simulink model "Basic_Drone_Waypoint_part"  (R2024a)
settings: Solver=FixedStepAuto  StartTime=0.0  StopTime=inf  FixedStep=0.1  RelTol=1e-3
undefined symbols (not defined in the file): Angle, Axis, DiscIntNeverNeededParam, gray
libraries: robotcorelib x10, slpidlib x4, eeGeneralControl x4, uavutilslib x1
settings Model: Creator=Sasha  LastModifiedBy=user

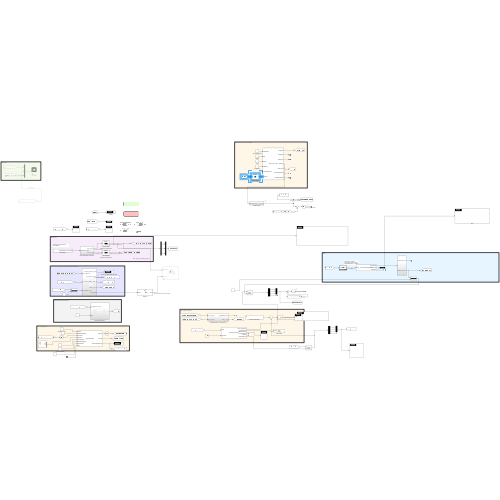
[thumbnail: Simulink's stored preview of the top-level diagram]
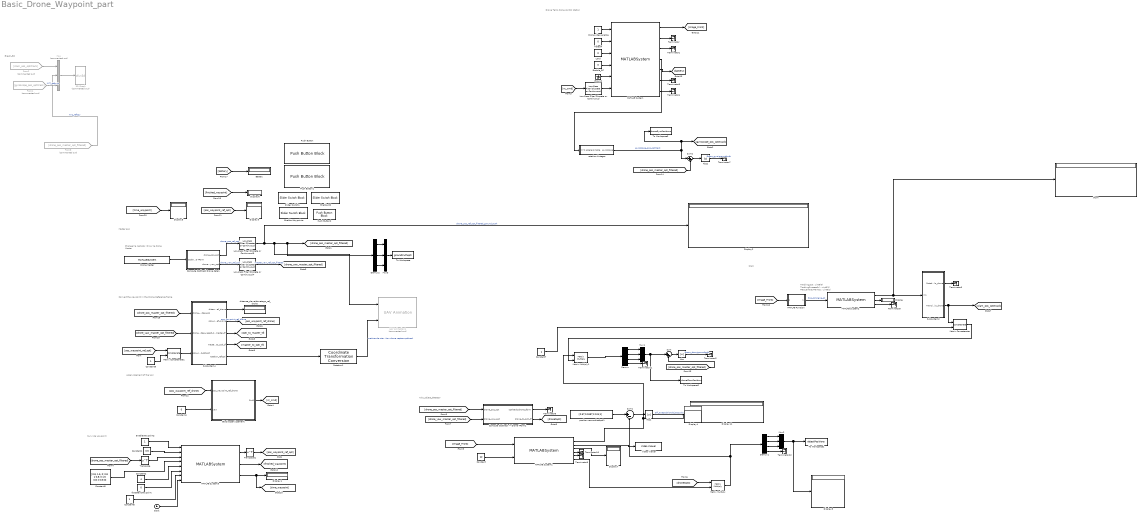
== system Basic_Drone_Waypoint_part ==
  note: Suivi de waypoint
  note: Drone Tello drone control station
  note: Asservissement of the UAV
  note: TrackingLost : uint8(0)
      | TrackingSuccessful : uint8(1)
      | FrequentKeyFrames : uint8(2)
  note: Slam
  note: Graph_3D
  note: Changer le rigibody ID sur le drone Master
  note: Master pos
  note: Convert the waypoint in the Drone Reference frame
  note: Yolo_object_detector
  3D Graph : S-Function  Commented=on  LoadFcn=if exist('sfun3d','file'), sfun3d([],[],[],'LoadBlock'); end  FunctionName=sfun3d  Parameters=ax,T,np,cp,gd,ls,mk,mx,hd,tb  SFunctionDeploymentMode=off  EnableBusSupport=off  mask(3D Graph){np=3, ax=[-5 5 -5 5 -5 5], mx=1e4, T=-1, cp=[3 2 1], gd=on, hd=off, tb=on, ls=-, mk=none}
      mask prompts: np "Number of moving points (lines)"; ax "Range: [xmin xmax  ymin ymax zmin zmax]"; mx "Max number of points in each line"; T "Sampling Time"; cp "Camera position (use [0 0 1] for 2D XY view)"; gd "Grid (on|off)"; hd "HeadMarkers (on|off)"; tb "Toolbar (on|off)"; ls "LineStyle"; mk "LineMarker"
      mask help:
      | This block plots the position of several points in the XYZ space. The input contains the coordinates of all the points (x1,y1,z1,x2,y2,z2,...).
      | The number of moving points (lines), the XYZ ranges, sampling time, camera position, and grid (among other things) can be set as mask parameters.
      settings: CopyFcn=if exist('sfun3d','file'), sfun3d([],[],[],'CopyBlock'); end  DeleteFcn=if exist('sfun3d','file'), sfun3d([],[],[],'DeleteBlock'); end  NameChangeFcn=if exist('sfun3d','file'), sfun3d([],[],[],'NameChange'); end
      mask Help:
      | This block plots the position of several points in the XYZ space. The input contains the coordinates of all the points (x1,y1,z1,x2,y2,z2,...).
      | The number of moving points (lines), the XYZ ranges, sampling time, camera position, and grid (among other things) can be set as mask parameters.
      mask TypeOptions ls: - | -- | : | -. | none
      mask TypeOptions mk: none | . | + | o | * | x | square | diamond | v | ^ | > | < | pentagram | hexagram
      mask Display: plot([.05 .95 .95 .05 .05],[.45 .45 .95 .95 .45], 0.5+cos(0:0.1:2*pi)*0.3,0.7+sin(0:0.1:2*pi)*0.2)
  Abs : Abs  SaturateOnIntegerOverflow=off
  Abs1 : Abs  SaturateOnIntegerOverflow=off
  Abs2 : Abs  SaturateOnIntegerOverflow=off
  Battery : Display
  "Block asservissement " : Subsystem
  Clock : Clock
  "Compute Optitrack -> Drone TForm1" : Subsystem
  Compute Optitrack Drone data1 : Subsystem
  Constant : Constant  Value=12
  Constant1 : Constant  Value=0.5
  Constant2 : Constant  Value=4
  Constant3 : Constant  Value=[0.8, 1.5, 0; 0.8 1 0.8; 0 1.5 0.8; 0 0.8 0]
  Constant4 : Constant  Value=0
  Constant5 : Constant
  Constant6 : Constant
  Constant7 : Constant
  Demux : Demux
  Demux1 : Demux
  Demux2 : Demux  Outputs=3
  Display{,1..8,11} (10 alike) : Display
  Drone Master : MATLABSystem  System=OptilinkSystem  HostIP=10.147.125.15  ClientIP=10.147.125.15  RigidbodyID=2  SimulateUsing=Interpreted execution
      mask Type: OptilinkSystem
      mask Display:
      | disp('OptilinkSystem');
      | port_label('output',1,'Drones data');
  Dronevideo enable : Constant
  Enable RC : SliderSwitchBlock
      settings: Values={{'Off', 'On'}, [0 1]}
  Enable Waypoints : SliderSwitchBlock
      settings: Values={{'Off', 'On'}, [0 1]}
  Enable_RC : Constant  Value=0
  From1 : From  Commented=on  GotoTag=gyroscope_pos_optitrack
  From2 : From  Commented=on  GotoTag=slam_pos_optitrack
  From8 : From  Commented=on  GotoTag=drone_pos_master_opt_filtered
  Ground : Ground
  Land : Constant  Value=0
  Low-Pass Filter (Discrete or Continuous) : eeGeneralControl/Low-Pass Filter (Discrete or Continuous)  K=1  T=1  B=inf  A=-inf  init_option=Inherited from block input  x0=0  Ts=-1
  Low-Pass Filter (Discrete or Continuous)4 : eeGeneralControl/Low-Pass Filter (Discrete or Continuous)  K=1  T=1.5  B=inf  A=-inf  init_option=Inherited from block input  x0=0  Ts=-1
  Low-Pass Filter (Discrete or Continuous)5 : eeGeneralControl/Low-Pass Filter (Discrete or Continuous)  K=1  T=1.5  B=inf  A=-inf  init_option=Inherited from block input  x0=0  Ts=-1
  MATLAB Function : MATLAB Function  TreatAsAtomicUnit=on
  MATLAB System : MATLABSystem  System=Tello_drone_control  droneIP=127.0.0.1  SimulateUsing=Interpreted execution
      mask Type: Tello_drone_control
      mask Display:
      | disp('Tello_drone_control');
      | port_label('input',1,'enableVideo');
      | port_label('input',2,'tkoff');
      | port_label('input',3,'landing');
      | port_label('input',4,'enableRC');
      | port_label('input',5,'cmdVideoDirection');
      | port_label('input',6,'rcspeeds');
      | port_label('output',1,'imageFront');
      | port_label('output',2,'imageDown');
      | port_label('output',3,'Eulerangles');
      | port_label('output',4,'speedXYZ');
      | port_label('output',5,'batteryLevel');
      | port_label('output',6,'currentVideoDirection');
      | port_label('output',7,'hasTakenOffStatus');
  MATLAB System1 : MATLABSystem  System=Yolo_Object_Detector  SimulateUsing=Interpreted execution
      mask Type: Yolo_Object_Detector
      mask Display:
      | disp('Yolo_Object_Detector');
      | port_label('input',1,'Image');
      | port_label('input',2,'degreecam');
      | port_label('output',1,'Tform_camtodrone');
      | port_label('output',2,'AnnotatedImage');
      | port_label('output',3,'BBoxDimensions');
      | port_label('output',4,'CamCoordinates');
      | port_label('output',5,'posecam');
      | port_label('output',6,'posecamtodrone');
  MATLAB System2 : MATLABSystem  System=MonoVisualSLAMSystem  FocalLength=[ 878, 883.00 ]  PrincipalPoint=[ 488, 363 ]  ImageSize=[ 720, 960 ]  ScaleFactor=1.2  NumLevels=6  MaxNumPoints=200  SkipMaxFrames=10  TrackFeatureRange=[ 50, 120 ]  LoopClosureThreshold=50  Verbose=false  ThreadLevel=3  SimulateUsing=Code generation
      mask Type: MonoVisualSLAMSystem
      mask Display:
      | disp('MonoVisualSLAMSystem');
      | port_label('input',1,'Image');
      | port_label('output',1,'Camera Pose');
      | port_label('output',2,'Tracking Lost');
      | port_label('output',3,'XYZ Points');
  MATLAB System3 : MATLABSystem  System=WaypointManager  SimulateUsing=Code generation
      mask Type: WaypointManager
      mask Display:
      | disp('WaypointManager');
      | port_label('input',1,'enable');
      | port_label('input',2,'lookaheadDistance');
      | port_label('input',3,'currentPos');
      | port_label('input',4,'waypoints');
      | port_label('input',5,'numWaypoints');
      | port_label('input',6,'forceNextWaypoint');
      | port_label('input',7,'requiredTime');
      | port_label('input',8,'time');
      | port_label('output',1,'waypoint');
      | port_label('output',2,'finished');
      | port_label('output',3,'elapsedTimeWaypoint');
  Matrix Concatenate : Concatenate  ConcatenateDimension=2
  Matrix Concatenate1 : Concatenate  ConcatenateDimension=2
  Matrix Multiply : Product  Multiplication=Matrix(*)
  Matrix Multiply1 : Product  Multiplication=Matrix(*)
  Mux : Mux  Commented=on  Inputs=3
  Mux1 : Mux  Inputs=3
  Mux2 : Mux  Inputs=3
  Mux3 : Mux  Inputs=3
  Push Button : PushButtonBlock  ButtonText=Décoler  OffValue=0.000000
  Push Button1 : PushButtonBlock  ButtonText=Atterir  OffValue=0.000000
  Push Button2 : PushButtonBlock  ButtonText=Next waypoint  OffValue=0.000000
  Rotation1 : robotcorelib/Coordinate Transformation Conversion  InputRepresentation=Rotation Matrix  InputEulerSequence=XYZ  ShowTrVecInputPort=off  OutputRepresentation=Quaternion  OutputEulerSequence=ZYX  ShowTrVecOutputPort=off  SimulateUsing=Code generation
      settings: LibrarySourceBlock=uavutilslib/Coordinate Transformation Conversion
  Slider Switch1 : SliderSwitchBlock
      settings: Values={{'Off', 'On'}, [0 1]}
  Subsystem2 : Subsystem
  Subsystem4 : Subsystem
  Sum : Sum  Inputs=|+-
  Sum1 : Sum  Inputs=|+-
  Sum2 : Sum  Inputs=|+-
  Takeoff : Constant  Value=0
  Terminator{,1..12} (13 alike) : Terminator
  To Workspace : ToWorkspace  VariableName=groundtruthopti  SampleTime=-1
  To Workspace1 : ToWorkspace  VariableName=objectPositions  SampleTime=-1
  To Workspace2 : ToWorkspace  VariableName=droneSlamPositions  SampleTime=-1
  To Workspace3 : ToWorkspace  VariableName=droneGyroPositions  SampleTime=-1
  Transpose : Math  Operator=transpose
  Transpose1 : Math  Operator=transpose
  UAV Animation1 : uavutilslib/UAV Animation  Commented=on  UAVType=Multirotor  UAVSize=1  InertialZDirection=Down  SampleTime=-1
  Video Viewer : VideoViewer  colormapValue=gray(256)  FigPos=[231 1060 894 657]
  distance_slave/slavetogo_ref_drone : Display
  enableWaypoints : Constant
  forceNextWaypoint : Constant  Value=0
  posiiton camordirefopti1 : Constant  Value=[0.57;0.1597;2.124;1]
  rotation+integer : Subsystem
  tform : Display
  wires:
  Land/1 -> MATLAB System/3
  Takeoff/1 -> MATLAB System/2
  Enable_RC/1 -> MATLAB System/4
  [rc_cmd] -> Low-Pass Filter (Discrete or Continuous)/1
  Low-Pass Filter (Discrete or Continuous)/1 -> MATLAB System/6
  MATLAB System/6 -> Terminator3/1
  MATLAB System2/2 -> Display/1
  MATLAB System2/1 -> tform/1, Subsystem2/1(In1)
  From8/1 -> Mux/2  "XYZ_refopy"
  Mux/1 -> 3D Graph/1
  From1/1 -> Mux/3  "XYZ_refgyro"
  MATLAB System/1 -> [Image_Front]
  MATLAB System/2 -> Terminator/1
  Dronevideo enable/1 -> MATLAB System/1
  MATLAB System/3 -> Terminator1/1
  MATLAB System/5 -> [battery]
  MATLAB System/7 -> Terminator4/1
  rotation+integer/1(gyroscope) -> [gyroscope_pos_optitrack], To Workspace3/1, Sum2/1  "gyroscope_pos_optitrack"
  Compute Optitrack Drone data1/1(drone_pos_opt) -> Low-Pass Filter (Discrete or Continuous)5/1  "drone_pos_ref_opt"
  Low-Pass Filter (Discrete or Continuous)4/1 -> [drone_yaw_master_opt_filtered]  "master_yaw_ref_opt_filtered"
  Compute Optitrack Drone data1/2(drone_yaw_opt) -> Low-Pass Filter (Discrete or Continuous)4/1  "drone_yaw_ref_opt"
  Low-Pass Filter (Discrete or Continuous)5/1 -> [drone_pos_master_opt_filtered], Demux2/1, UAV Animation1/1, Display2/1  "drone_pos_ref_opt_filtered_ground_truth"
  Drone Master/1 -> Compute Optitrack Drone data1/1(Optitrack Drone TForm)
  [drone_yaw_master_opt_filtered] -> Subsystem4/2(drone_master_yaw)
  Subsystem4/1(distance_waypoint_ref_drone) -> distance_slave/slavetogo_ref_drone/1
  Subsystem4/2(pos_waypoint_ref_drone) -> [pos_waypoint_ref_drone]  "pos_waypoint_ref_drone"
  [drone_pos_master_opt_filtered] -> Subsystem4/1(drone_master_pos)
  "Block asservissement "/1(Out1) -> [rc_cmd]
  Ground/1 -> MATLAB System/5
  Constant4/1 -> "Block asservissement "/2(yaw)
  MATLAB System2/3 -> Terminator5/1
  [pos_waypoint_ref_opt] -> Matrix Concatenate1/1
  [Image_Front] -> MATLAB Function/1(inputImage)
  MATLAB Function/1(grayImage) -> MATLAB System2/1  "Pos_consigne_pt"
  Subsystem4/3(opti_to_master_tf) -> [opti_to_master_tf]
  Subsystem4/4(master_to_opti_tf) -> [master_to_opti_tf]
  Sum/1 -> Abs/1
  Abs/1 -> Terminator2/1  "Erreur_slam/groundtruth"
  [drone_pos_master_opt_filtered] -> Sum2/2
  Sum2/1 -> Abs2/1
  Abs2/1 -> Terminator7/1  "Erreur_gyro/groundtruth"
  [drone_pos_master_opt_filtered] -> Sum/2
  Mux1/1 -> To Workspace2/1, Sum/1
  Subsystem2/2(Translation Tello_drone) -> Matrix Concatenate/1, [slam_pos_optitrack]
  enableWaypoints/1 -> MATLAB System3/1
  Constant1/1 -> MATLAB System3/2
  Constant3/1 -> MATLAB System3/4
  Constant2/1 -> MATLAB System3/5
  forceNextWaypoint/1 -> MATLAB System3/6
  MATLAB System3/1 -> Transpose1/1
  [pos_waypoint_ref_drone] -> "Block asservissement "/1(pos_waypoint_ref_drone)
  Transpose1/1 -> [pos_waypoint_ref_opt]
  Matrix Concatenate1/1 -> Subsystem4/3(pos_waypoint_ref_opt)
  Constant5/1 -> Matrix Concatenate1/2
  [pos_waypoint_ref_opt] -> Display3/1
  MATLAB System3/2 -> [finished_waypoint]
  [finished_waypoint] -> Display6/1
  [battery] -> Battery/1
  Constant6/1 -> MATLAB System3/7
  Clock/1 -> MATLAB System3/8
  [drone_pos_master_opt_filtered] -> Transpose/1
  Transpose/1 -> MATLAB System3/3
  MATLAB System3/3 -> [time_waypoint], Display1/1
  Constant/1 -> MATLAB System1/2
  Abs1/1 -> Display4/1  "Dif_truepositionobj/posyolo"
  [drone_pos_master_opt_filtered] -> "Compute Optitrack -> Drone TForm1"/1(drone_pos_opt)
  [dronetopti] -> Matrix Multiply/1
  MATLAB System1/3 -> Display7/1
  posiiton camordirefopti1/1 -> Sum1/1
  MATLAB System1/6 -> Matrix Multiply/2
  [drone_yaw_master_opt_filtered] -> "Compute Optitrack -> Drone TForm1"/2(drone_yaw_opt)
  "Compute Optitrack -> Drone TForm1"/1(optitrack2drone_tform) -> Terminator8/1
  "Compute Optitrack -> Drone TForm1"/2(drone_to_opti_tf) -> [dronetopti]
  Sum1/1 -> Abs1/1
  MATLAB System1/2 -> Video Viewer/1
  [Image_Front] -> MATLAB System1/1
  MATLAB System1/1 -> Matrix Multiply1/1, Display11/1
  MATLAB System1/5 -> Terminator9/1
  MATLAB System1/4 -> Terminator10/1
  Matrix Multiply1/1 -> Demux/1
  Constant7/1 -> Matrix Concatenate/2
  Matrix Concatenate/1 -> Matrix Multiply1/2
  Demux/2 -> Mux1/2
  Demux/1 -> Mux1/1
  Demux/3 -> Mux1/3
  Demux/4 -> Terminator11/1
  From2/1 -> Mux/1
  Subsystem4/5(rotation_refopti) -> Rotation1/1
  Rotation1/1 -> UAV Animation1/2  "matrice de rotation drone repère optitrack"
  [time_waypoint] -> Display5/1
  Demux1/3 -> Mux2/3
  Demux1/2 -> Mux2/2
  Matrix Multiply/1 -> Demux1/1, Sum1/2
  Mux2/1 -> Display8/1, To Workspace1/1
  Demux1/4 -> Terminator12/1
  Demux1/1 -> Mux2/1
  MATLAB System/4 -> rotation+integer/1(XYZ acceleromètre)
  Demux2/3 -> Mux3/3
  Demux2/1 -> Mux3/1
  Mux3/1 -> To Workspace/1
  Demux2/2 -> Mux3/2
  Subsystem2/1(Rotation Tello_drone) -> Terminator6/1

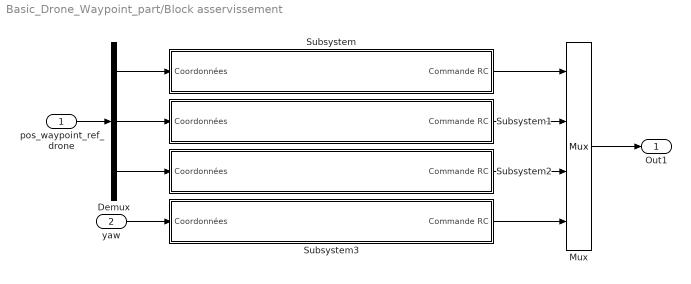
== system Basic_Drone_Waypoint_part/Block asservissement  ==
  pos_waypoint_ref_drone : Inport
  yaw : Inport  Port=2
  Demux : Demux  Outputs=3
  Mux : Mux
  Subsystem : Subsystem
  Subsystem1 : Subsystem
  Subsystem2 : Subsystem
  Subsystem3 : Subsystem
  Out1 : Outport
  wires:
  pos_waypoint_ref_drone/1 -> Demux/1
  Mux/1 -> Out1/1
  Demux/1 -> Subsystem/1(Coordonnées)
  Subsystem/1(Commande RC) -> Mux/1
  Subsystem1/1(Commande RC) -> Mux/2
  Demux/2 -> Subsystem1/1(Coordonnées)
  Demux/3 -> Subsystem2/1(Coordonnées)
  Subsystem2/1(Commande RC) -> Mux/3
  yaw/1 -> Subsystem3/1(Coordonnées)
  Subsystem3/1(Commande RC) -> Mux/4

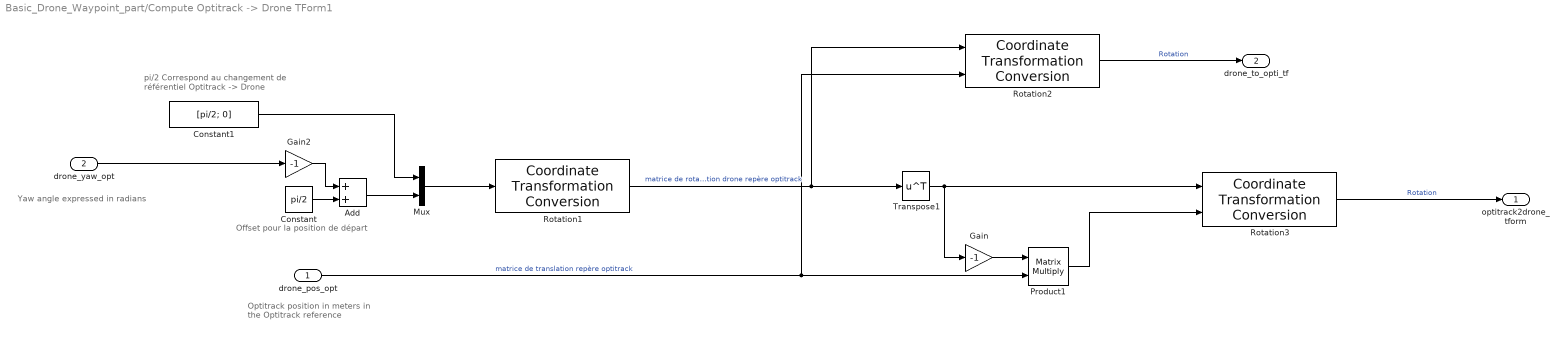
== system Basic_Drone_Waypoint_part/Compute Optitrack -> Drone TForm1 ==
  note: Yaw angle expressed in radians
  note: Offset pour la position de départ
  note: pi/2 Correspond au changement de référentiel Optitrack -> Drone
  note: Optitrack position in meters
      | in the Optitrack reference
  drone_pos_opt : Inport
  drone_yaw_opt : Inport  Port=2
  Add : Sum
  Constant : Constant  Value=pi/2
  Constant1 : Constant  Value=[pi/2; 0]
  Gain : Gain  Gain=-1
  Gain2 : Gain  Gain=-1
  Mux : Mux  Inputs=2
  Product1 : Product  Multiplication=Matrix(*)
  Rotation1 : robotcorelib/Coordinate Transformation Conversion  InputRepresentation=Euler Angles  InputEulerSequence=XYZ  ShowTrVecInputPort=off  OutputRepresentation=Rotation Matrix  OutputEulerSequence=ZYX  ShowTrVecOutputPort=off  SimulateUsing=Code generation
      settings: LibrarySourceBlock=uavutilslib/Coordinate Transformation Conversion
  Rotation2 : robotcorelib/Coordinate Transformation Conversion  InputRepresentation=Rotation Matrix  InputEulerSequence=XYZ  ShowTrVecInputPort=on  OutputRepresentation=Homogeneous Transformation  OutputEulerSequence=ZYX  ShowTrVecOutputPort=off  SimulateUsing=Code generation
      settings: LibrarySourceBlock=uavutilslib/Coordinate Transformation Conversion
  Rotation3 : robotcorelib/Coordinate Transformation Conversion  InputRepresentation=Rotation Matrix  InputEulerSequence=XYZ  ShowTrVecInputPort=on  OutputRepresentation=Homogeneous Transformation  OutputEulerSequence=ZYX  ShowTrVecOutputPort=off  SimulateUsing=Code generation
      settings: LibrarySourceBlock=uavutilslib/Coordinate Transformation Conversion
  Transpose1 : Math  Operator=transpose
  optitrack2drone_tform : Outport
  drone_to_opti_tf : Outport  Port=2
  wires:
  Add/1 -> Mux/2
  Transpose1/1 -> Rotation3/1, Gain/1
  Constant/1 -> Add/2
  Gain2/1 -> Add/1
  Product1/1 -> Rotation3/2
  Constant1/1 -> Mux/1
  Rotation1/1 -> Rotation2/1, Transpose1/1  "matrice de rotation drone repère optitrack"
  Gain/1 -> Product1/1
  Mux/1 -> Rotation1/1
  drone_pos_opt/1 -> Rotation2/2, Product1/2  "matrice de translation repère optitrack"
  drone_yaw_opt/1 -> Gain2/1
  Rotation3/1 -> optitrack2drone_tform/1  "Rotation"
  Rotation2/1 -> drone_to_opti_tf/1  "Rotation"

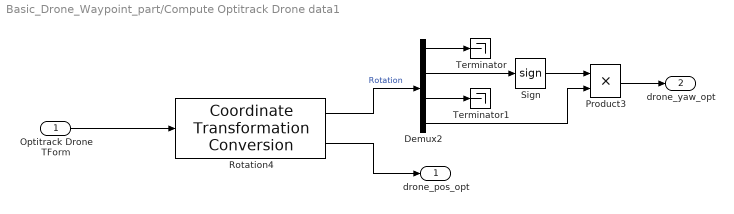
== system Basic_Drone_Waypoint_part/Compute Optitrack Drone data1 ==
  Optitrack Drone TForm : Inport
  Demux2 : Demux
  Product3 : Product
  Rotation4 : robotcorelib/Coordinate Transformation Conversion  InputRepresentation=Homogeneous Transformation  InputEulerSequence=XYZ  ShowTrVecInputPort=on  OutputRepresentation=Axis-Angle  OutputEulerSequence=XYZ  ShowTrVecOutputPort=on  SimulateUsing=Code generation
      settings: LibrarySourceBlock=uavutilslib/Coordinate Transformation Conversion
  Sign : Signum
  Terminator : Terminator
  Terminator1 : Terminator
  drone_pos_opt : Outport
  drone_yaw_opt : Outport  Port=2
  wires:
  Rotation4/2 -> drone_pos_opt/1
  Demux2/4 -> Product3/2
  Rotation4/1 -> Demux2/1  "Rotation"
  Sign/1 -> Product3/1
  Demux2/2 -> Sign/1
  Product3/1 -> drone_yaw_opt/1
  Optitrack Drone TForm/1 -> Rotation4/1
  Demux2/3 -> Terminator1/1
  Demux2/1 -> Terminator/1

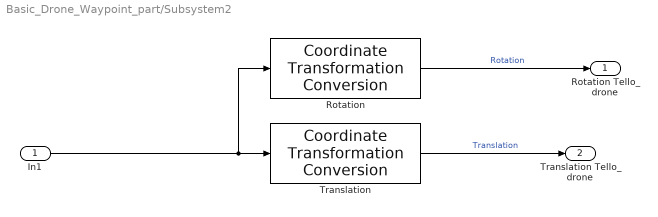
== system Basic_Drone_Waypoint_part/Subsystem2 ==
  In1 : Inport
  Rotation : robotcorelib/Coordinate Transformation Conversion  InputRepresentation=Homogeneous Transformation  InputEulerSequence=ZYX  ShowTrVecInputPort=on  OutputRepresentation=Quaternion  OutputEulerSequence=ZYX  ShowTrVecOutputPort=off  SimulateUsing=Code generation
      settings: LibrarySourceBlock=uavutilslib/Coordinate Transformation Conversion
  Translation : robotcorelib/Coordinate Transformation Conversion  InputRepresentation=Homogeneous Transformation  InputEulerSequence=ZYX  ShowTrVecInputPort=on  OutputRepresentation=Translation Vector  OutputEulerSequence=ZYX  ShowTrVecOutputPort=on  SimulateUsing=Code generation
      settings: LibrarySourceBlock=uavutilslib/Coordinate Transformation Conversion
  Rotation Tello_drone : Outport
  Translation Tello_drone : Outport  Port=2
  wires:
  Translation/1 -> Translation Tello_drone/1  "Translation"
  Rotation/1 -> Rotation Tello_drone/1  "Rotation"
  In1/1 -> Rotation/1, Translation/1

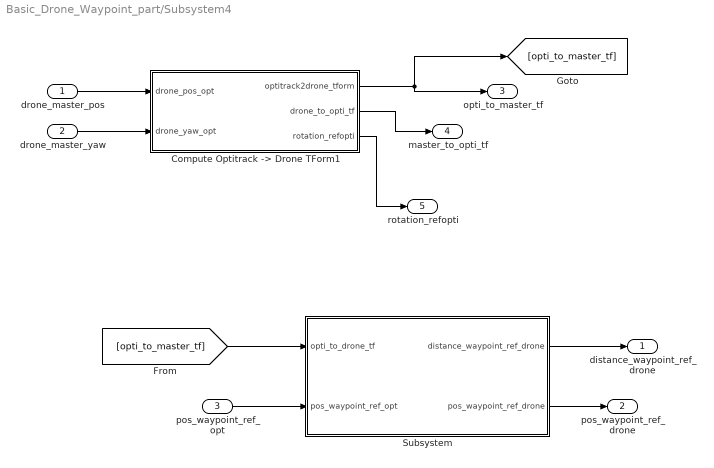
== system Basic_Drone_Waypoint_part/Subsystem4 ==
  drone_master_pos : Inport
  drone_master_yaw : Inport  Port=2
  pos_waypoint_ref_opt : Inport  Port=3
  "Compute Optitrack -> Drone TForm1" : Subsystem
  Subsystem : Subsystem
  distance_waypoint_ref_drone : Outport
  pos_waypoint_ref_drone : Outport  Port=2
  opti_to_master_tf : Outport  Port=3
  master_to_opti_tf : Outport  Port=4
  rotation_refopti : Outport  Port=5
  wires:
  Subsystem/1(distance_waypoint_ref_drone) -> distance_waypoint_ref_drone/1
  Subsystem/2(pos_waypoint_ref_drone) -> pos_waypoint_ref_drone/1
  drone_master_pos/1 -> "Compute Optitrack -> Drone TForm1"/1(drone_pos_opt)
  drone_master_yaw/1 -> "Compute Optitrack -> Drone TForm1"/2(drone_yaw_opt)
  "Compute Optitrack -> Drone TForm1"/2(drone_to_opti_tf) -> master_to_opti_tf/1
  [opti_to_master_tf] -> Subsystem/1(opti_to_drone_tf)
  pos_waypoint_ref_opt/1 -> Subsystem/2(pos_waypoint_ref_opt)
  "Compute Optitrack -> Drone TForm1"/1(optitrack2drone_tform) -> opti_to_master_tf/1, [opti_to_master_tf]
  "Compute Optitrack -> Drone TForm1"/3(rotation_refopti) -> rotation_refopti/1

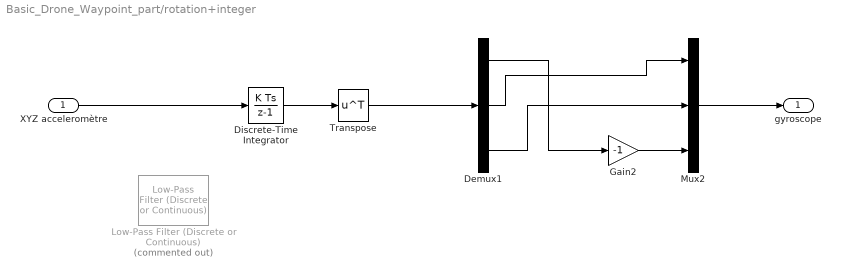
== system Basic_Drone_Waypoint_part/rotation+integer ==
  XYZ acceleromètre : Inport
  Demux1 : Demux  Outputs=3
  Discrete-Time Integrator : DiscreteIntegrator  SampleTime=-1  ICPrevOutput=DiscIntNeverNeededParam  ICPrevScaledInput=DiscIntNeverNeededParam
  Gain2 : Gain  Gain=-1
  Low-Pass Filter (Discrete or Continuous) : eeGeneralControl/Low-Pass Filter (Discrete or Continuous)  Commented=on  K=1  T=1  B=inf  A=-inf  init_option=Inherited from block input  x0=0  Ts=-1
  Mux2 : Mux  Inputs=3
  Transpose : Math  Operator=transpose
  gyroscope : Outport
  wires:
  Discrete-Time Integrator/1 -> Transpose/1
  Mux2/1 -> gyroscope/1
  Demux1/3 -> Mux2/2
  Demux1/2 -> Mux2/1
  Gain2/1 -> Mux2/3
  Demux1/1 -> Gain2/1
  Transpose/1 -> Demux1/1
  XYZ acceleromètre/1 -> Discrete-Time Integrator/1

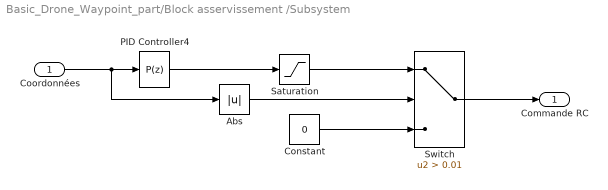
== system Basic_Drone_Waypoint_part/Block asservissement /Subsystem ==
  Coordonnées : Inport
  Abs : Abs  SaturateOnIntegerOverflow=off
  Constant : Constant  Value=0
  PID Controller4 : slpidlib/PID Controller  Controller=P  Form=Parallel  TimeDomain=Discrete-time  UseExternalTs=off  SampleTime=-1  IntegratorMethod=Forward Euler  FilterMethod=Forward Euler  ControllerParametersSource=internal  P=45  I=0.0168470505938331  UseKiTs=off  D=0.181138103439247  UseExternalDerivativeSource=off  N=1.15322702769143  UseFilter=on  TunerSelectOption=Transfer Function Based (PID Tuner App)  InitialConditionSource=internal  InitialConditionForIntegrator=0  InitialConditionForFilter=0  DifferentiatorICPrevScaledInput=0  ExternalReset=none  TrackingMode=off  Kt=1  LimitOutput=off  SatLimitsSource=internal  UpperSaturationLimit=inf  LowerSaturationLimit=-inf  LinearizeAsGain=on  AntiWindupMode=none  Kb=1  LimitIntegrator=on  UpperIntegratorSaturationLimit=0.5  LowerIntegratorSaturationLimit=-0.5  POutMin=[]  POutMax=[]  IOutMin=[]  IOutMax=[]  DOutMin=[]  DOutMax=[]  NOutMin=[]  NOutMax=[]  SumOutMin=[]  SumOutMax=[]  SaturationOutMin=[]  SaturationOutMax=[]  PParamMin=[]  PParamMax=[]  IParamMin=[]  IParamMax=[]  DParamMin=[]  DParamMax=[]  NParamMin=[]  NParamMax=[]  KbParamMin=[]  KbParamMax=[]  KtParamMin=[]  KtParamMax=[]  KbOutMin=[]  KbOutMax=[]  KtOutMin=[]  KtOutMax=[]  IntegratorOutMin=[]  IntegratorOutMax=[]  FilterOutMin=[]  FilterOutMax=[]  SumI1OutMin=[]  SumI1OutMax=[]  SumI2OutMin=[]  SumI2OutMax=[]  SumI3OutMin=[]  SumI3OutMax=[]  SumI4OutMin=[]  SumI4OutMax=[]  SumDOutMin=[]  SumDOutMax=[]  DifferentiatorOutMin=[]  DifferentiatorOutMax=[]  FilterDiffOutCoefMin=[]  FilterDiffOutCoefMax=[]  ReciprocalOutMin=[]  ReciprocalOutMax=[]  SumDenOutMin=[]  SumDenOutMax=[]  SumNumOutMin=[]  SumNumOutMax=[]  DivideOutMin=[]  DivideOutMax=[]  UdiffTsProdOutMin=[]  UdiffTsProdOutMax=[]  NTsProdOutMin=[]  NTsProdOutMax=[]  UintegralTsProdOutMin=[]  UintegralTsProdOutMax=[]  UngainTsProdOutMin=[]  UngainTsProdOutMax=[]  ClampingZeroOutDataTypeStr=Inherit: Inherit via back propagation  ClampingZeroOutMin=[]  ClampingZeroOutMax=[]  FilterDenConstantOutDataTypeStr=Inherit: Inherit via back propagation  FilterDenConstantOutMin=[]  FilterDenConstantOutMax=[]  PCopyOutDataTypeStr=Inherit: Inherit via back propagation  PCopyOutMin=[]  PCopyOutMax=[]  NCopyOutDataTypeStr=Inherit: Inherit via back propagation  NCopyOutMin=[]  NCopyOutMax=[]  IntegratorContinuousStateAttributes=''  IntegratorStateMustResolveToSignalObject=off  IntegratorRTWStateStorageClass=Auto  FilterContinuousStateAttributes=''  FilterStateMustResolveToSignalObject=off  FilterRTWStateStorageClass=Auto  ParallelPVariant=InternalParameters  IdealPVariant=Disabled  IVariant=Disabled  DVariant=Disabled  IntegratorVariant=Disabled  SatVariant=Disabled  AWVariant=Disabled  PCopyVariant=Disabled  TRVariant=Disabled  FdbkBlocksVariant=Forward  IdealPFdbkVariant=Disabled  SatFdbkVariant=Disabled  DerivativeFilterVariant=Disabled  NVariant=Disabled  NCopyVariant=Disabled_SignalSpec  FilterICVariant=Disabled  IntegratorICVariant=Disabled  ExternalResetVariant=Disabled  TRSumVariant=Passthrough  SumFdbkVariant=Disabled  SumVariant=Passthrough_P  TsampFilterVariant=InternalTs  TsampNgainVariant=Passthrough  TsampIntegralVariant=Disabled_SignalSpec  ExternalSaturationOutDataTypeStr=Inherit: Same as second input  DerivativeSourceVariant=Disabled
  Saturation : Saturate  UpperLimit=20  LowerLimit=-20
  Switch : Switch  Criteria=u2 > Threshold  Threshold=0.01  SaturateOnIntegerOverflow=off  InputSameDT=off
  Commande RC : Outport
  wires:
  PID Controller4/1 -> Saturation/1
  Coordonnées/1 -> Abs/1, PID Controller4/1
  Saturation/1 -> Switch/1
  Constant/1 -> Switch/3
  Switch/1 -> Commande RC/1
  Abs/1 -> Switch/2

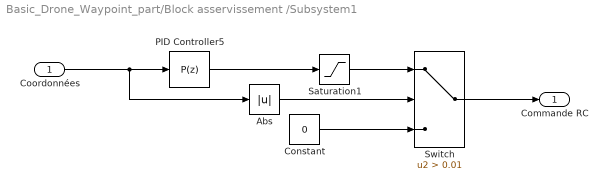
== system Basic_Drone_Waypoint_part/Block asservissement /Subsystem1 ==
  Coordonnées : Inport
  Abs : Abs  SaturateOnIntegerOverflow=off
  Constant : Constant  Value=0
  PID Controller5 : slpidlib/PID Controller  Controller=P  Form=Parallel  TimeDomain=Discrete-time  UseExternalTs=off  SampleTime=-1  IntegratorMethod=Forward Euler  FilterMethod=Forward Euler  ControllerParametersSource=internal  P=45  I=0.0168470505938331  UseKiTs=off  D=0.181138103439247  UseExternalDerivativeSource=off  N=1.15322702769143  UseFilter=on  TunerSelectOption=Transfer Function Based (PID Tuner App)  InitialConditionSource=internal  InitialConditionForIntegrator=0  InitialConditionForFilter=0  DifferentiatorICPrevScaledInput=0  ExternalReset=none  TrackingMode=off  Kt=1  LimitOutput=off  SatLimitsSource=internal  UpperSaturationLimit=inf  LowerSaturationLimit=-inf  LinearizeAsGain=on  AntiWindupMode=none  Kb=1  LimitIntegrator=on  UpperIntegratorSaturationLimit=0.5  LowerIntegratorSaturationLimit=-0.5  POutMin=[]  POutMax=[]  IOutMin=[]  IOutMax=[]  DOutMin=[]  DOutMax=[]  NOutMin=[]  NOutMax=[]  SumOutMin=[]  SumOutMax=[]  SaturationOutMin=[]  SaturationOutMax=[]  PParamMin=[]  PParamMax=[]  IParamMin=[]  IParamMax=[]  DParamMin=[]  DParamMax=[]  NParamMin=[]  NParamMax=[]  KbParamMin=[]  KbParamMax=[]  KtParamMin=[]  KtParamMax=[]  KbOutMin=[]  KbOutMax=[]  KtOutMin=[]  KtOutMax=[]  IntegratorOutMin=[]  IntegratorOutMax=[]  FilterOutMin=[]  FilterOutMax=[]  SumI1OutMin=[]  SumI1OutMax=[]  SumI2OutMin=[]  SumI2OutMax=[]  SumI3OutMin=[]  SumI3OutMax=[]  SumI4OutMin=[]  SumI4OutMax=[]  SumDOutMin=[]  SumDOutMax=[]  DifferentiatorOutMin=[]  DifferentiatorOutMax=[]  FilterDiffOutCoefMin=[]  FilterDiffOutCoefMax=[]  ReciprocalOutMin=[]  ReciprocalOutMax=[]  SumDenOutMin=[]  SumDenOutMax=[]  SumNumOutMin=[]  SumNumOutMax=[]  DivideOutMin=[]  DivideOutMax=[]  UdiffTsProdOutMin=[]  UdiffTsProdOutMax=[]  NTsProdOutMin=[]  NTsProdOutMax=[]  UintegralTsProdOutMin=[]  UintegralTsProdOutMax=[]  UngainTsProdOutMin=[]  UngainTsProdOutMax=[]  ClampingZeroOutDataTypeStr=Inherit: Inherit via back propagation  ClampingZeroOutMin=[]  ClampingZeroOutMax=[]  FilterDenConstantOutDataTypeStr=Inherit: Inherit via back propagation  FilterDenConstantOutMin=[]  FilterDenConstantOutMax=[]  PCopyOutDataTypeStr=Inherit: Inherit via back propagation  PCopyOutMin=[]  PCopyOutMax=[]  NCopyOutDataTypeStr=Inherit: Inherit via back propagation  NCopyOutMin=[]  NCopyOutMax=[]  IntegratorContinuousStateAttributes=''  IntegratorStateMustResolveToSignalObject=off  IntegratorRTWStateStorageClass=Auto  FilterContinuousStateAttributes=''  FilterStateMustResolveToSignalObject=off  FilterRTWStateStorageClass=Auto  ParallelPVariant=InternalParameters  IdealPVariant=Disabled  IVariant=Disabled  DVariant=Disabled  IntegratorVariant=Disabled  SatVariant=Disabled  AWVariant=Disabled  PCopyVariant=Disabled  TRVariant=Disabled  FdbkBlocksVariant=Forward  IdealPFdbkVariant=Disabled  SatFdbkVariant=Disabled  DerivativeFilterVariant=Disabled  NVariant=Disabled  NCopyVariant=Disabled_SignalSpec  FilterICVariant=Disabled  IntegratorICVariant=Disabled  ExternalResetVariant=Disabled  TRSumVariant=Passthrough  SumFdbkVariant=Disabled  SumVariant=Passthrough_P  TsampFilterVariant=InternalTs  TsampNgainVariant=Passthrough  TsampIntegralVariant=Disabled_SignalSpec  ExternalSaturationOutDataTypeStr=Inherit: Same as second input  DerivativeSourceVariant=Disabled
  Saturation1 : Saturate  UpperLimit=20  LowerLimit=-20
  Switch : Switch  Criteria=u2 > Threshold  Threshold=0.01  SaturateOnIntegerOverflow=off  InputSameDT=off
  Commande RC : Outport
  wires:
  Constant/1 -> Switch/3
  Switch/1 -> Commande RC/1
  PID Controller5/1 -> Saturation1/1
  Coordonnées/1 -> Abs/1, PID Controller5/1
  Saturation1/1 -> Switch/1
  Abs/1 -> Switch/2

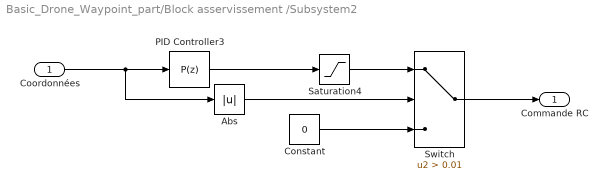
== system Basic_Drone_Waypoint_part/Block asservissement /Subsystem2 ==
  Coordonnées : Inport
  Abs : Abs  SaturateOnIntegerOverflow=off
  Constant : Constant  Value=0
  PID Controller3 : slpidlib/PID Controller  Controller=P  Form=Parallel  TimeDomain=Discrete-time  UseExternalTs=off  SampleTime=-1  IntegratorMethod=Forward Euler  FilterMethod=Forward Euler  ControllerParametersSource=internal  P=-37.5  I=0.0168470505938331  UseKiTs=off  D=0.181138103439247  UseExternalDerivativeSource=off  N=1.15322702769143  UseFilter=on  TunerSelectOption=Transfer Function Based (PID Tuner App)  InitialConditionSource=internal  InitialConditionForIntegrator=0  InitialConditionForFilter=0  DifferentiatorICPrevScaledInput=0  ExternalReset=none  TrackingMode=off  Kt=1  LimitOutput=off  SatLimitsSource=internal  UpperSaturationLimit=inf  LowerSaturationLimit=-inf  LinearizeAsGain=on  AntiWindupMode=none  Kb=1  LimitIntegrator=on  UpperIntegratorSaturationLimit=0.5  LowerIntegratorSaturationLimit=-0.5  POutMin=[]  POutMax=[]  IOutMin=[]  IOutMax=[]  DOutMin=[]  DOutMax=[]  NOutMin=[]  NOutMax=[]  SumOutMin=[]  SumOutMax=[]  SaturationOutMin=[]  SaturationOutMax=[]  PParamMin=[]  PParamMax=[]  IParamMin=[]  IParamMax=[]  DParamMin=[]  DParamMax=[]  NParamMin=[]  NParamMax=[]  KbParamMin=[]  KbParamMax=[]  KtParamMin=[]  KtParamMax=[]  KbOutMin=[]  KbOutMax=[]  KtOutMin=[]  KtOutMax=[]  IntegratorOutMin=[]  IntegratorOutMax=[]  FilterOutMin=[]  FilterOutMax=[]  SumI1OutMin=[]  SumI1OutMax=[]  SumI2OutMin=[]  SumI2OutMax=[]  SumI3OutMin=[]  SumI3OutMax=[]  SumI4OutMin=[]  SumI4OutMax=[]  SumDOutMin=[]  SumDOutMax=[]  DifferentiatorOutMin=[]  DifferentiatorOutMax=[]  FilterDiffOutCoefMin=[]  FilterDiffOutCoefMax=[]  ReciprocalOutMin=[]  ReciprocalOutMax=[]  SumDenOutMin=[]  SumDenOutMax=[]  SumNumOutMin=[]  SumNumOutMax=[]  DivideOutMin=[]  DivideOutMax=[]  UdiffTsProdOutMin=[]  UdiffTsProdOutMax=[]  NTsProdOutMin=[]  NTsProdOutMax=[]  UintegralTsProdOutMin=[]  UintegralTsProdOutMax=[]  UngainTsProdOutMin=[]  UngainTsProdOutMax=[]  ClampingZeroOutDataTypeStr=Inherit: Inherit via back propagation  ClampingZeroOutMin=[]  ClampingZeroOutMax=[]  FilterDenConstantOutDataTypeStr=Inherit: Inherit via back propagation  FilterDenConstantOutMin=[]  FilterDenConstantOutMax=[]  PCopyOutDataTypeStr=Inherit: Inherit via back propagation  PCopyOutMin=[]  PCopyOutMax=[]  NCopyOutDataTypeStr=Inherit: Inherit via back propagation  NCopyOutMin=[]  NCopyOutMax=[]  IntegratorContinuousStateAttributes=''  IntegratorStateMustResolveToSignalObject=off  IntegratorRTWStateStorageClass=Auto  FilterContinuousStateAttributes=''  FilterStateMustResolveToSignalObject=off  FilterRTWStateStorageClass=Auto  ParallelPVariant=InternalParameters  IdealPVariant=Disabled  IVariant=Disabled  DVariant=Disabled  IntegratorVariant=Disabled  SatVariant=Disabled  AWVariant=Disabled  PCopyVariant=Disabled  TRVariant=Disabled  FdbkBlocksVariant=Forward  IdealPFdbkVariant=Disabled  SatFdbkVariant=Disabled  DerivativeFilterVariant=Disabled  NVariant=Disabled  NCopyVariant=Disabled_SignalSpec  FilterICVariant=Disabled  IntegratorICVariant=Disabled  ExternalResetVariant=Disabled  TRSumVariant=Passthrough  SumFdbkVariant=Disabled  SumVariant=Passthrough_P  TsampFilterVariant=InternalTs  TsampNgainVariant=Passthrough  TsampIntegralVariant=Disabled_SignalSpec  ExternalSaturationOutDataTypeStr=Inherit: Same as second input  DerivativeSourceVariant=Disabled
  Saturation4 : Saturate  UpperLimit=20  LowerLimit=-20
  Switch : Switch  Criteria=u2 > Threshold  Threshold=0.01  SaturateOnIntegerOverflow=off  InputSameDT=off
  Commande RC : Outport
  wires:
  Constant/1 -> Switch/3
  Switch/1 -> Commande RC/1
  PID Controller3/1 -> Saturation4/1
  Coordonnées/1 -> Abs/1, PID Controller3/1
  Saturation4/1 -> Switch/1
  Abs/1 -> Switch/2

== system Basic_Drone_Waypoint_part/Block asservissement /Subsystem3 ==
  Coordonnées : Inport
  Gain3 : Gain  Gain=20
  PID Controller1 : slpidlib/PID Controller  Controller=P  Form=Parallel  TimeDomain=Continuous-time  UseExternalTs=off  SampleTime=-1  IntegratorMethod=Forward Euler  FilterMethod=Forward Euler  ControllerParametersSource=internal  P=3  I=0.0168470505938331  UseKiTs=off  D=0.181138103439247  UseExternalDerivativeSource=off  N=1.15322702769143  UseFilter=on  TunerSelectOption=Transfer Function Based (PID Tuner App)  InitialConditionSource=internal  InitialConditionForIntegrator=0  InitialConditionForFilter=0  DifferentiatorICPrevScaledInput=0  ExternalReset=none  TrackingMode=off  Kt=1  LimitOutput=off  SatLimitsSource=internal  UpperSaturationLimit=inf  LowerSaturationLimit=-inf  LinearizeAsGain=on  AntiWindupMode=none  Kb=1  LimitIntegrator=on  UpperIntegratorSaturationLimit=0.5  LowerIntegratorSaturationLimit=-0.5  POutMin=[]  POutMax=[]  IOutMin=[]  IOutMax=[]  DOutMin=[]  DOutMax=[]  NOutMin=[]  NOutMax=[]  SumOutMin=[]  SumOutMax=[]  SaturationOutMin=[]  SaturationOutMax=[]  PParamMin=[]  PParamMax=[]  IParamMin=[]  IParamMax=[]  DParamMin=[]  DParamMax=[]  NParamMin=[]  NParamMax=[]  KbParamMin=[]  KbParamMax=[]  KtParamMin=[]  KtParamMax=[]  KbOutMin=[]  KbOutMax=[]  KtOutMin=[]  KtOutMax=[]  IntegratorOutMin=[]  IntegratorOutMax=[]  FilterOutMin=[]  FilterOutMax=[]  SumI1OutMin=[]  SumI1OutMax=[]  SumI2OutMin=[]  SumI2OutMax=[]  SumI3OutMin=[]  SumI3OutMax=[]  SumI4OutMin=[]  SumI4OutMax=[]  SumDOutMin=[]  SumDOutMax=[]  DifferentiatorOutMin=[]  DifferentiatorOutMax=[]  FilterDiffOutCoefMin=[]  FilterDiffOutCoefMax=[]  ReciprocalOutMin=[]  ReciprocalOutMax=[]  SumDenOutMin=[]  SumDenOutMax=[]  SumNumOutMin=[]  SumNumOutMax=[]  DivideOutMin=[]  DivideOutMax=[]  UdiffTsProdOutMin=[]  UdiffTsProdOutMax=[]  NTsProdOutMin=[]  NTsProdOutMax=[]  UintegralTsProdOutMin=[]  UintegralTsProdOutMax=[]  UngainTsProdOutMin=[]  UngainTsProdOutMax=[]  ClampingZeroOutDataTypeStr=Inherit: Inherit via back propagation  ClampingZeroOutMin=[]  ClampingZeroOutMax=[]  FilterDenConstantOutDataTypeStr=Inherit: Inherit via back propagation  FilterDenConstantOutMin=[]  FilterDenConstantOutMax=[]  PCopyOutDataTypeStr=Inherit: Inherit via back propagation  PCopyOutMin=[]  PCopyOutMax=[]  NCopyOutDataTypeStr=Inherit: Inherit via back propagation  NCopyOutMin=[]  NCopyOutMax=[]  IntegratorContinuousStateAttributes=''  IntegratorStateMustResolveToSignalObject=off  IntegratorRTWStateStorageClass=Auto  FilterContinuousStateAttributes=''  FilterStateMustResolveToSignalObject=off  FilterRTWStateStorageClass=Auto  ParallelPVariant=InternalParameters  IdealPVariant=Disabled  IVariant=Disabled  DVariant=Disabled  IntegratorVariant=Disabled  SatVariant=Disabled  AWVariant=Disabled  PCopyVariant=Disabled  TRVariant=Disabled  FdbkBlocksVariant=Forward  IdealPFdbkVariant=Disabled  SatFdbkVariant=Disabled  DerivativeFilterVariant=Disabled  NVariant=Disabled  NCopyVariant=Disabled_SignalSpec  FilterICVariant=Disabled  IntegratorICVariant=Disabled  ExternalResetVariant=Disabled  TRSumVariant=Passthrough  SumFdbkVariant=Disabled  SumVariant=Passthrough_P  TsampFilterVariant=InternalTs  TsampNgainVariant=Passthrough  TsampIntegralVariant=Disabled_SignalSpec  ExternalSaturationOutDataTypeStr=Inherit: Same as second input  DerivativeSourceVariant=Disabled
  Saturation3 : Saturate  UpperLimit=50  LowerLimit=-50
  Commande RC : Outport
  wires:
  Saturation3/1 -> Commande RC/1
  Gain3/1 -> Saturation3/1
  PID Controller1/1 -> Gain3/1
  Coordonnées/1 -> PID Controller1/1

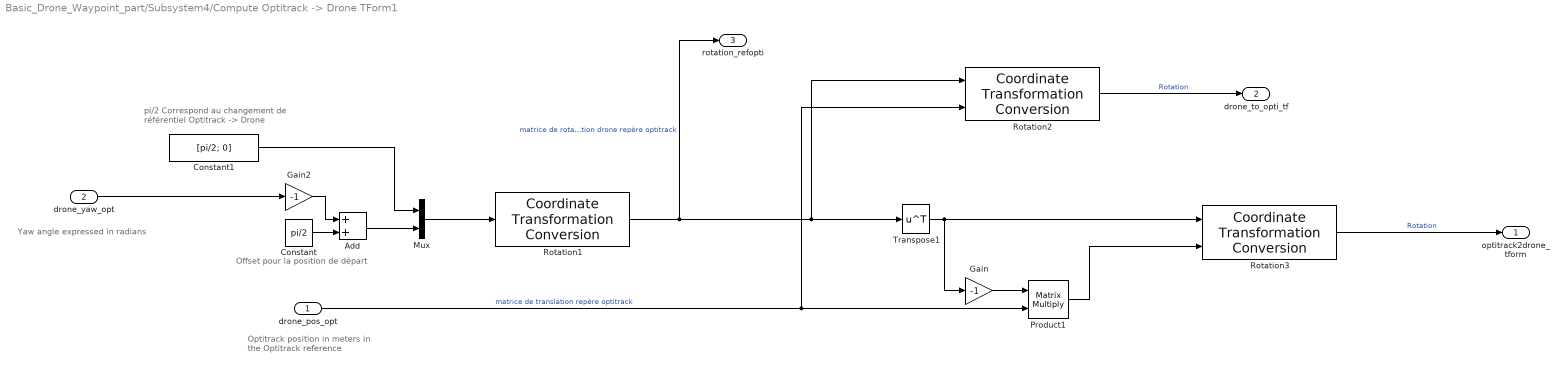
== system Basic_Drone_Waypoint_part/Subsystem4/Compute Optitrack -> Drone TForm1 ==
  note: Yaw angle expressed in radians
  note: Offset pour la position de départ
  note: pi/2 Correspond au changement de référentiel Optitrack -> Drone
  note: Optitrack position in meters
      | in the Optitrack reference
  drone_pos_opt : Inport
  drone_yaw_opt : Inport  Port=2
  Add : Sum
  Constant : Constant  Value=pi/2
  Constant1 : Constant  Value=[pi/2; 0]
  Gain : Gain  Gain=-1
  Gain2 : Gain  Gain=-1
  Mux : Mux  Inputs=2
  Product1 : Product  Multiplication=Matrix(*)
  Rotation1 : robotcorelib/Coordinate Transformation Conversion  InputRepresentation=Euler Angles  InputEulerSequence=XYZ  ShowTrVecInputPort=off  OutputRepresentation=Rotation Matrix  OutputEulerSequence=ZYX  ShowTrVecOutputPort=off  SimulateUsing=Code generation
      settings: LibrarySourceBlock=uavutilslib/Coordinate Transformation Conversion
  Rotation2 : robotcorelib/Coordinate Transformation Conversion  InputRepresentation=Rotation Matrix  InputEulerSequence=XYZ  ShowTrVecInputPort=on  OutputRepresentation=Homogeneous Transformation  OutputEulerSequence=ZYX  ShowTrVecOutputPort=off  SimulateUsing=Code generation
      settings: LibrarySourceBlock=uavutilslib/Coordinate Transformation Conversion
  Rotation3 : robotcorelib/Coordinate Transformation Conversion  InputRepresentation=Rotation Matrix  InputEulerSequence=XYZ  ShowTrVecInputPort=on  OutputRepresentation=Homogeneous Transformation  OutputEulerSequence=ZYX  ShowTrVecOutputPort=off  SimulateUsing=Code generation
      settings: LibrarySourceBlock=uavutilslib/Coordinate Transformation Conversion
  Transpose1 : Math  Operator=transpose
  optitrack2drone_tform : Outport
  drone_to_opti_tf : Outport  Port=2
  rotation_refopti : Outport  Port=3
  wires:
  Add/1 -> Mux/2
  Transpose1/1 -> Rotation3/1, Gain/1
  Constant/1 -> Add/2
  Gain2/1 -> Add/1
  Product1/1 -> Rotation3/2
  Constant1/1 -> Mux/1
  Rotation1/1 -> rotation_refopti/1, Rotation2/1, Transpose1/1  "matrice de rotation drone repère optitrack"
  Gain/1 -> Product1/1
  Mux/1 -> Rotation1/1
  drone_pos_opt/1 -> Rotation2/2, Product1/2  "matrice de translation repère optitrack"
  drone_yaw_opt/1 -> Gain2/1
  Rotation3/1 -> optitrack2drone_tform/1  "Rotation"
  Rotation2/1 -> drone_to_opti_tf/1  "Rotation"

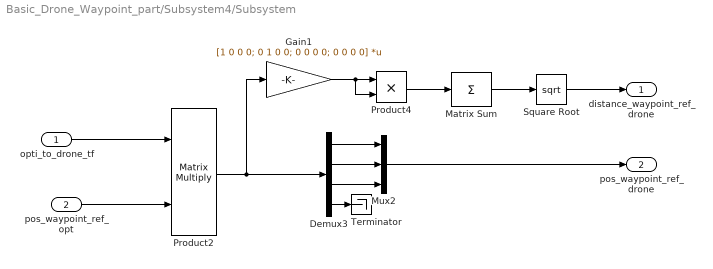
== system Basic_Drone_Waypoint_part/Subsystem4/Subsystem ==
  opti_to_drone_tf : Inport
  pos_waypoint_ref_opt : Inport  Port=2
  Demux3 : Demux
  Gain1 : Gain  Gain=[1 0 0 0; 0 1 0 0; 0 0 0 0; 0 0 0 0]  Multiplication=Matrix(K*u)
  Matrix Sum : Sum  Inputs=+
  Mux2 : Mux  Inputs=3
  Product2 : Product  Multiplication=Matrix(*)
  Product4 : Product
  Square Root : Sqrt
  Terminator : Terminator
  distance_waypoint_ref_drone : Outport
  pos_waypoint_ref_drone : Outport  Port=2
  wires:
  Product2/1 -> Gain1/1, Demux3/1
  opti_to_drone_tf/1 -> Product2/1
  Product4/1 -> Matrix Sum/1
  Demux3/2 -> Mux2/2
  Square Root/1 -> distance_waypoint_ref_drone/1
  Demux3/1 -> Mux2/1
  Gain1/1 -> Product4/2, Product4/1
  Matrix Sum/1 -> Square Root/1
  Demux3/3 -> Mux2/3
  Demux3/4 -> Terminator/1
  pos_waypoint_ref_opt/1 -> Product2/2
  Mux2/1 -> pos_waypoint_ref_drone/1

== matlab function Basic_Drone_Waypoint_part/MATLAB Function ==
  data: inputImage input; grayImage output
function grayImage = convertToGrayscale(inputImage)
    % Convert the input image to grayscale
        grayImage = rgb2gray(inputImage);
end
